simulink model "simulink_model"  (R2018a)
settings: Solver=VariableStepAuto  StartTime=0.0  StopTime=0.06  RelTol=1e-3
libraries: simulink x1
settings Model: Creator=hp  LastModifiedBy=hp

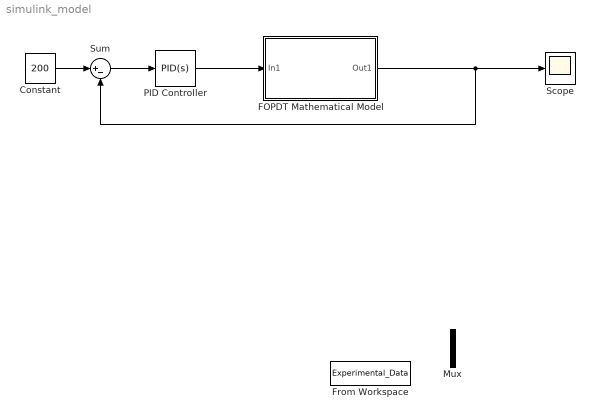
== system simulink_model ==
  Constant : Constant  Value=200
  "FOPDT Mathematical Model " : Subsystem
  From Workspace : FromWorkspace  VariableName=Experimental_Data  SampleTime=0
  Mux : Mux  Inputs=2
  PID Controller : simulink/Continuous/PID Controller  Controller=PID  TimeDomain=Continuous-time  SampleTime=-1  IntegratorMethod=Forward Euler  FilterMethod=Forward Euler  Form=Parallel  UseFilter=on  ControllerParametersSource=internal  P=-1.61689974469037  I=-22600.3881462445  D=8.39692052001722e-06  N=26440.151411389  InitialConditionSource=internal  InitialConditionForIntegrator=0  InitialConditionForFilter=0  ExternalReset=none  LimitOutput=off  UpperSaturationLimit=inf  LowerSaturationLimit=-inf  LinearizeAsGain=on  AntiWindupMode=none  Kb=1  TrackingMode=off  Kt=1  PParamMin=[]  PParamMax=[]  IParamMin=[]  IParamMax=[]  DParamMin=[]  DParamMax=[]  NParamMin=[]  NParamMax=[]  KbParamMin=[]  KbParamMax=[]  KtParamMin=[]  KtParamMax=[]  POutMin=[]  POutMax=[]  IOutMin=[]  IOutMax=[]  DOutMin=[]  DOutMax=[]  NOutMin=[]  NOutMax=[]  KbOutMin=[]  KbOutMax=[]  KtOutMin=[]  KtOutMax=[]  IntegratorOutMin=[]  IntegratorOutMax=[]  FilterOutMin=[]  FilterOutMax=[]  SumOutMin=[]  SumOutMax=[]  SumI1OutMin=[]  SumI1OutMax=[]  SumI2OutMin=[]  SumI2OutMax=[]  SumI3OutMin=[]  SumI3OutMax=[]  SumDOutMin=[]  SumDOutMax=[]  SaturationOutMin=[]  SaturationOutMax=[]  IntegratorContinuousStateAttributes=''  IntegratorStateMustResolveToSignalObject=off  IntegratorRTWStateStorageClass=Auto  FilterContinuousStateAttributes=''  FilterStateMustResolveToSignalObject=off  FilterRTWStateStorageClass=Auto  DifferentiatorICPrevScaledInput=0  DifferentiatorOutMin=[]  DifferentiatorOutMax=[]  FilterDiffOutCoefMin=[]  FilterDiffOutCoefMax=[]  SumDenOutMin=[]  SumDenOutMax=[]  SumNumOutMin=[]  SumNumOutMax=[]  ReciprocalOutMin=[]  ReciprocalOutMax=[]  DivideOutMin=[]  DivideOutMax=[]  TunerSelectOption=Transfer Function Based (PID Tuner App)
  Scope : Scope
  Sum : Sum  Inputs=|+-
  wires:
  "FOPDT Mathematical Model "/1(Out1) -> Sum/2, Scope/1
  PID Controller/1 -> "FOPDT Mathematical Model "/1(In1)
  Sum/1 -> PID Controller/1
  Constant/1 -> Sum/1

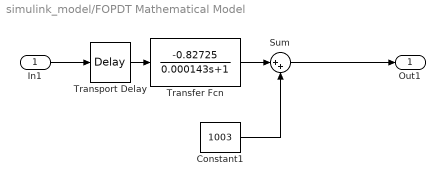
== system simulink_model/FOPDT Mathematical Model  ==
  In1 : Inport
  Constant1 : Constant  Value=1003
  Sum : Sum  Inputs=|++
  Transfer Fcn : TransferFcn  Numerator=[-0.82725]  Denominator=[0.000143 1]
  Transport Delay : TransportDelay  DelayTime=0
  Out1 : Outport
  wires:
  In1/1 -> Transport Delay/1
  Constant1/1 -> Sum/2
  Transfer Fcn/1 -> Sum/1
  Sum/1 -> Out1/1
  Transport Delay/1 -> Transfer Fcn/1
